simulink model "main_sim_noadapt"  (Simulink 7.2)
settings: Solver=ode2  SolverMode=SingleTasking  StartTime=0.0  StopTime=tsim_max  FixedStep=dtsim  RelTol=1e-3
StopFcn:
  | %mkplt
values from neighbouring files (symbols this model uses):
  vel = 128    [do_command_tracking.m]
undefined symbols (not defined in the file or in its folder): accel_cmd, aero_surf_qbar_off, aero_surf_qbar_on, assertion_time, att_cmd_select, att_trim_IC, att_type, att_type_numbers, bb_ellipsoid, bb_params, chi_trim_IC, command_time, compute_all_rate_cols, compute_all_vel_cols, constants, cosA, da_trim_IC, dc_L2W_IC, de_trim_IC, DiscIntNeverNeededParam, dr_trim_IC, dtsim, E_rwy, E_trim_IC, Ed_cmd, Ed_trim_IC, eow_boundary, flag_exsig, full_surf_llim, full_surf_ulim, gain_set, gain_var_struct, gam_cmd_descent, gam_cmd_preflare, gamdot_cmd_descent, gamdot_cmd_flare, gamdot_cmd_preflare, gamma_trim_IC, h_trim_IC, hd_cmd, hd_trim_IC, ideal_vel_Kb, in_exsig_vecin, in_exsig_vecout, in_t_exsig, MACH, MACH_att_fb, MACH_att_int_IC, MACH_att_Kb, MACH_att_Kc, MACH_att_Ki, MACH_gain_mat, MACH_mass_IC, MACH_pos_IC, MACH_pos_int_IC, MACH_pos_Kb, MACH_pos_Kc, MACH_pos_Ki, MACH_pqr_Bmat_IC, MACH_pqr_IC ... (+62)
libraries: simulink x36, utility_lib x34, mach_lib x24, model_lib x13, simulink_need_slupdate x8, models x8
(part 3 of 7)

== system main_sim_noadapt/claw_main/state est/process inputs ==
  u_old : Inport  OutDataType=sfix(16)  OutScaling=2^0
  sensors : Inport  Port=2  OutDataType=sfix(16)  OutScaling=2^0
  Bus Selector2 : BusSelector  OutputSignals=u_meas
  Constant : Constant  Value=0  OutDataType=sfix(16)  OutScaling=2^0
  Multiport Switch1 : MultiPortSwitch  Inputs=2  zeroidx=on  SaturateOnIntegerOverflow=on
  throt : Selector  InputPortWidth=MACH.num_u  IndexOptions=Index vector (dialog)  Indices=MACH.throttle_idx  OutputSizes=1
  use throt estimate from measurement instead of past throt cmd : Assignment  IndexOptions=Index vector (dialog)  Indices=MACH.throttle_idx  OutputSizes=[1 1]
  use_throt_estimate : Constant  Value=use_throt_estimate  OutDataType=sfix(16)  OutScaling=2^0
  zero RCS inputs : Assignment  IndexOptions=Index vector (dialog)  Indices=MACH.rcs_idx  OutputSizes=[1 1]
  u_est : Outport  OutDataType=sfix(16)  OutScaling=2^0
  wires:
  u_old/1 -> use throt estimate from measurement instead of past throt cmd/1, Multiport Switch1/2
  use_throt_estimate/1 -> Multiport Switch1/1
  use throt estimate from measurement instead of past throt cmd/1 -> Multiport Switch1/3
  sensors/1 -> Bus Selector2/1
  Bus Selector2/1 -> throt/1  "<u_meas>"
  Multiport Switch1/1 -> zero RCS inputs/1
  Constant/1 -> zero RCS inputs/2
  zero RCS inputs/1 -> u_est/1
  throt/1 -> use throt estimate from measurement instead of past throt cmd/2

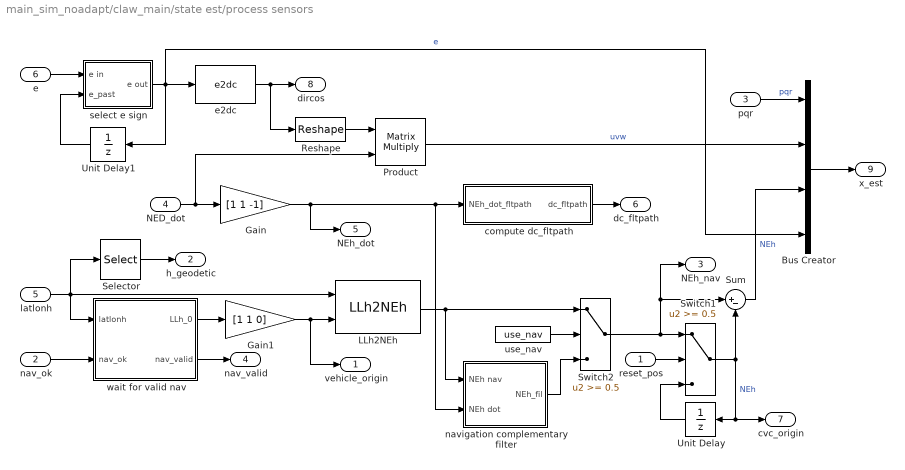
== system main_sim_noadapt/claw_main/state est/process sensors ==
  reset_pos : Inport  OutDataType=sfix(16)  OutScaling=2^0
  nav_ok : Inport  Port=2  OutDataType=sfix(16)  OutScaling=2^0
  pqr : Inport  Port=3  OutDataType=sfix(16)  OutScaling=2^0
  NED_dot : Inport  Port=4  OutDataType=sfix(16)  OutScaling=2^0
  latlonh : Inport  Port=5  OutDataType=sfix(16)  OutScaling=2^0
  e : Inport  Port=6  OutDataType=sfix(16)  OutScaling=2^0
  Bus Creator : BusCreator
  Gain : Gain  Gain=[1 1 -1]  ParameterDataType=sfix(16)  ParameterScaling=2^0  OutDataType=sfix(16)  OutScaling=2^0  SaturateOnIntegerOverflow=on  OutDataTypeStr=Inherit: Same as input  ParamDataTypeStr=Inherit: Same as input
  Gain1 : Gain  Gain=[1 1 0]  ParameterDataType=sfix(16)  ParameterScaling=2^0  OutDataType=sfix(16)  OutScaling=2^0  SaturateOnIntegerOverflow=on  OutDataTypeStr=Inherit: Same as input  ParamDataTypeStr=Inherit: Same as input
  LLh2NEh : utility_lib/LLh2NEh  SystemSampleTime=-1
  Product : Product  Multiplication=Matrix(*)  OutDataType=sfix(16)  OutScaling=2^0  SaturateOnIntegerOverflow=on  OutDataTypeStr=Inherit: Same as first input
  Reshape : Reshape  OutputDimensionality=Customize  OutputDimensions=[3,3]
  Selector : Selector  InputPortWidth=3  IndexOptions=Index vector (dialog)  Indices=[3]  OutputSizes=1
  Sum : Sum  Inputs=|+-  OutDataType=sfix(16)  OutScaling=2^0  SaturateOnIntegerOverflow=on
  Switch1 : Switch  Threshold=0.5  SaturateOnIntegerOverflow=on
  Switch2 : Switch  Threshold=0.5  SaturateOnIntegerOverflow=on
  Unit Delay : UnitDelay  Orientation=left  SampleTime=-1
  Unit Delay1 : UnitDelay  Orientation=left  X0=MACH_quat_IC  SampleTime=-1
  compute dc_fltpath : Subsystem
  e2dc : utility_lib/e2dc  SystemSampleTime=-1
  navigation complementary filter : Subsystem
  select e sign : Subsystem
  use_nav : Constant  Value=use_nav  OutDataType=sfix(16)  OutScaling=2^0
  wait for valid nav : Subsystem
  vehicle_origin : Outport  OutDataType=sfix(16)  OutScaling=2^0
  h_geodetic : Outport  Port=2  OutDataType=sfix(16)  OutScaling=2^0
  NEh_nav : Outport  Port=3  OutDataType=sfix(16)  OutScaling=2^0
  nav_valid : Outport  Port=4  OutDataType=sfix(16)  OutScaling=2^0
  NEh_dot : Outport  Port=5  OutDataType=sfix(16)  OutScaling=2^0
  dc_fltpath : Outport  Port=6  OutDataType=sfix(16)  OutScaling=2^0
  cvc_origin : Outport  Port=7  OutDataType=sfix(16)  OutScaling=2^0
  dircos : Outport  Port=8  OutDataType=sfix(16)  OutScaling=2^0
  x_est : Outport  Port=9  OutDataType=sfix(16)  OutScaling=2^0
  wires:
  e/1 -> select e sign/1(e in)
  Unit Delay1/1 -> select e sign/2(e_past)
  wait for valid nav/1(LLh_0) -> Gain1/1
  Sum/1 -> Bus Creator/3  "NEh"
  navigation complementary filter/1(NEh_fil) -> Switch2/3
  use_nav/1 -> Switch2/2
  Switch2/1 -> Sum/1, NEh_nav/1, Switch1/1
  Unit Delay/1 -> Switch1/3
  Switch1/1 -> Unit Delay/1, cvc_origin/1, Sum/2  "NEh"
  LLh2NEh/1 -> navigation complementary filter/1(NEh nav), Switch2/1
  wait for valid nav/2(nav_valid) -> nav_valid/1
  nav_ok/1 -> wait for valid nav/2(nav_ok)
  reset_pos/1 -> Switch1/2
  latlonh/1 -> wait for valid nav/1(latlonh), LLh2NEh/1, Selector/1
  e2dc/1 -> dircos/1, Reshape/1
  NED_dot/1 -> Product/2, Gain/1
  Gain/1 -> navigation complementary filter/2(NEh dot), compute dc_fltpath/1(NEh_dot_fltpath), NEh_dot/1
  select e sign/1(e out) -> Unit Delay1/1, e2dc/1, Bus Creator/4  "e"
  Reshape/1 -> Product/1
  pqr/1 -> Bus Creator/1  "pqr"
  Product/1 -> Bus Creator/2  "uvw"
  Bus Creator/1 -> x_est/1
  Selector/1 -> h_geodetic/1
  Gain1/1 -> LLh2NEh/2, vehicle_origin/1
  compute dc_fltpath/1(dc_fltpath) -> dc_fltpath/1

== system main_sim_noadapt/claw_main/state est/wind estimator ==
  dircos : Inport  OutDataType=sfix(16)  OutScaling=2^0
  x : Inport  Port=2  OutDataType=sfix(16)  OutScaling=2^0
  sensors : Inport  Port=3  OutDataType=sfix(16)  OutScaling=2^0
  u : Inport  Port=4  OutDataType=sfix(16)  OutScaling=2^0
  wind_est_sw : Inport  Port=5  OutDataType=sfix(16)  OutScaling=2^0
  Bus Selector1 : BusSelector  OutputSignals=NED_wind,accels_cg
  Bus Selector2 : BusSelector  OutputSignals=accels_cg
  Multiport Switch1 : MultiPortSwitch  Inputs=2  zeroidx=on  SaturateOnIntegerOverflow=on
  Unit Delay : UnitDelay  X0=zeros(3,1)  SampleTime=-1
  cl model : models/gtm-obac  SystemSampleTime=-1
  use_wind_est : Constant  Value=use_wind_est  OutDataType=sfix(16)  OutScaling=2^0
  wind estimate : Subsystem
  w_est : Outport  OutDataType=sfix(16)  OutScaling=2^0
  w_est_debug : Outport  Port=2  OutDataType=sfix(16)  OutScaling=2^0
  wires:
  cl model/1 -> wind estimate/3(xdot)
  Unit Delay/1 -> cl model/3
  use_wind_est/1 -> Multiport Switch1/1
  wind estimate/1(w_est) -> Unit Delay/1, Multiport Switch1/3
  x/1 -> wind estimate/2(x), cl model/1
  u/1 -> cl model/2
  dircos/1 -> wind estimate/1(dircos)
  Multiport Switch1/1 -> w_est/1
  wind_est_sw/1 -> wind estimate/6(wind_est_sw)
  sensors/1 -> Bus Selector1/1
  wind estimate/2(w_est_debug) -> w_est_debug/1
  Bus Selector1/1 -> Multiport Switch1/2  "<NED_wind>"
  Bus Selector1/2 -> wind estimate/5(sensed_accels_cg)  "<accels_cg>"
  cl model/2 -> Bus Selector2/1
  Bus Selector2/1 -> wind estimate/4(model_accels_cg)  "<accels_cg>"

== system main_sim_noadapt/claw_main/vel_loops/B matrix comp ==
  note: Note: Ideally,  X_nom and U_nom
      |  would be constructed to be near
      |  moment equalibrium
  X : Inport  OutDataType=sfix(16)  OutScaling=2^0
  U_limited : Inport  Port=2  OutDataType=sfix(16)  OutScaling=2^0
  d_nom : Inport  Port=3  OutDataType=sfix(16)  OutScaling=2^0
  camcmd : Inport  Port=4  OutDataType=sfix(16)  OutScaling=2^0
  params : Inport  Port=5  OutDataType=sfix(16)  OutScaling=2^0
  w_est : Inport  Port=6  OutDataType=sfix(16)  OutScaling=2^0
  NEh_dot : Inport  Port=7  OutDataType=sfix(16)  OutScaling=2^0
  scoped_bus : Inport  Port=8  OutDataType=sfix(16)  OutScaling=2^0
  B matrix comp : Subsystem  TreatAsAtomicUnit=on
  Constant : Constant  Value=0  OutDataType=sfix(16)  OutScaling=2^0
  Constant1 : Constant  Value=0  OutDataType=sfix(16)  OutScaling=2^0
  compute cvd_nom : Subsystem
  compute nominal XU : Subsystem
  zero pqr : Assignment  IndexOptions=Index vector (dialog)  Indices=MACH.pqr_idx  OutputSizes=[1 1]
  zero rate surfs : Assignment  IndexOptions=Index vector (dialog)  Indices=MACH.pqr_u_idx  OutputSizes=[1 1]
  cvd_nom : Outport  OutDataType=sfix(16)  OutScaling=2^0
  Bmat : Outport  Port=2  OutDataType=sfix(16)  OutScaling=2^0
  wires:
  camcmd/1 -> B matrix comp/6(camcmd), compute nominal XU/4(camcmd)
  scoped_bus/1 -> B matrix comp/9(scoped_bus)
  d_nom/1 -> B matrix comp/5(d_nom), compute nominal XU/3(D_in)
  params/1 -> B matrix comp/8(params)
  NEh_dot/1 -> B matrix comp/7(NEh_dot), compute nominal XU/5(NEh_dot)
  compute cvd_nom/1(cvd) -> cvd_nom/1, B matrix comp/1(cvd_nom)
  w_est/1 -> B matrix comp/4(w_est), compute cvd_nom/3(w_est)
  B matrix comp/1(Bmat) -> Bmat/1
  compute nominal XU/1(X_out) -> compute cvd_nom/1(x), B matrix comp/2(X_nom)
  compute nominal XU/2(U_out) -> compute cvd_nom/2(u), B matrix comp/3(U_nom)
  zero rate surfs/1 -> compute nominal XU/2(U_in)
  zero pqr/1 -> compute nominal XU/1(X_in)
  Constant/1 -> zero pqr/2
  Constant1/1 -> zero rate surfs/2
  U_limited/1 -> zero rate surfs/1
  X/1 -> zero pqr/1

== system main_sim_noadapt/claw_main/vel_loops/compute trim ==
  inner cmd : Inport  OutDataType=sfix(16)  OutScaling=2^0
  Bmat : Inport  Port=2  OutDataType=sfix(16)  OutScaling=2^0
  cmd : Inport  Port=3  OutDataType=sfix(16)  OutScaling=2^0
  Product : Product  Multiplication=Matrix(*)  OutDataType=sfix(16)  OutScaling=2^0  SaturateOnIntegerOverflow=on  OutDataTypeStr=Inherit: Same as first input
  Sum1 : Sum  Inputs=|+-  OutDataType=sfix(16)  OutScaling=2^0  SaturateOnIntegerOverflow=on
  trim : Outport  OutDataType=sfix(16)  OutScaling=2^0
  wires:
  Product/1 -> trim/1
  Bmat/1 -> Product/1
  Sum1/1 -> Product/2
  inner cmd/1 -> Sum1/1
  cmd/1 -> Sum1/2

== system main_sim_noadapt/claw_main/vel_loops/config_di ==
  cvd_nom : Inport  OutDataType=sfix(16)  OutScaling=2^0
  Bmat : Inport  Port=2  OutDataType=sfix(16)  OutScaling=2^0
  d_old : Inport  Port=3  OutDataType=sfix(16)  OutScaling=2^0
  d_nom : Inport  Port=4  OutDataType=sfix(16)  OutScaling=2^0
  cvd_des : Inport  Port=5  OutDataType=sfix(16)  OutScaling=2^0
  params : Inport  Port=6  OutDataType=sfix(16)  OutScaling=2^0
  di_smn : mach_lib/di_smn  SystemSampleTime=-1
  d_cmd : Outport  OutDataType=sfix(16)  OutScaling=2^0
  cvd_extra : Outport  Port=2  OutDataType=sfix(16)  OutScaling=2^0
  lambda : Outport  Port=3  OutDataType=sfix(16)  OutScaling=2^0
  solve_dat : Outport  Port=4  OutDataType=sfix(16)  OutScaling=2^0
  wires:
  cvd_nom/1 -> di_smn/1
  Bmat/1 -> di_smn/2
  d_old/1 -> di_smn/3
  d_nom/1 -> di_smn/4
  cvd_des/1 -> di_smn/5
  params/1 -> di_smn/6
  di_smn/1 -> d_cmd/1
  di_smn/2 -> cvd_extra/1
  di_smn/3 -> lambda/1
  di_smn/4 -> solve_dat/1

== system main_sim_noadapt/claw_main/vel_loops/convert accel_cmd to NED_dd_cmd ==
  accel_cmd : Inport  OutDataType=sfix(16)  OutScaling=2^0
  accel_cmd_sw : Inport  Port=2  OutDataType=sfix(16)  OutScaling=2^0
  NEh_d : Inport  Port=3  OutDataType=sfix(16)  OutScaling=2^0
  Merge : Merge  InitialOutput=zeros(3,1)
  MinMax : MinMax  Function=max  OutDataType=sfix(16)  OutScaling=2^0
  NED_dd cmd : Subsystem  TreatAsAtomicUnit=on
  Switch Case : SwitchCase  CaseConditions={1,2}  CaseShowDefault=off
  vchigam_dot cmd : Subsystem  TreatAsAtomicUnit=on
  NEh_dd_cmd : Outport  OutDataType=sfix(16)  OutScaling=2^0
  wires:
  accel_cmd_sw/1 -> MinMax/1
  MinMax/1 -> Switch Case/1
  NEh_d/1 -> vchigam_dot cmd/2(NEh_d)
  vchigam_dot cmd/1(NEh_dd_cmd) -> Merge/2
  Merge/1 -> NEh_dd_cmd/1
  Switch Case/1 -> NED_dd cmd/Action
  Switch Case/2 -> vchigam_dot cmd/Action
  accel_cmd/1 -> vchigam_dot cmd/1(vchigam_dot_cmd), NED_dd cmd/1(NEH_dd_cmd_in)
  NED_dd cmd/1(NEh_dd_cmd) -> Merge/1

== system main_sim_noadapt/claw_main/vel_loops/from inner ==
  att,T : Inport  OutDataType=sfix(16)  OutScaling=2^0
  Demux1 : Demux  Outputs=[ 2 1 MACH.num_u_throt ]
  Mux1 : Mux  Inputs=2
  Terminator : Terminator
  d_cmd : Outport  OutDataType=sfix(16)  OutScaling=2^0
  wires:
  att,T/1 -> Demux1/1
  Demux1/1 -> Mux1/1
  Mux1/1 -> d_cmd/1
  Demux1/3 -> Mux1/2
  Demux1/2 -> Terminator/1

== system main_sim_noadapt/claw_main/vel_loops/from quat ==
  e,T : Inport  OutDataType=sfix(16)  OutScaling=2^0
  Demux1 : Demux  Outputs=[ 4 MACH.num_u_throt ]
  Mux1 : Mux  Inputs=2
  Selector1 : Selector  InputPortWidth=3  IndexOptions=Index vector (dialog)  Indices=1:2  OutputSizes=1
  e2att : utility_lib/e2att  SystemSampleTime=-1
  d_cmd : Outport  OutDataType=sfix(16)  OutScaling=2^0
  wires:
  e2att/1 -> Selector1/1
  Selector1/1 -> Mux1/1
  Demux1/2 -> Mux1/2
  Mux1/1 -> d_cmd/1
  Demux1/1 -> e2att/1
  e,T/1 -> Demux1/1

== system main_sim_noadapt/claw_main/vel_loops/select vel cmd ==
  NEh_dot_current : Inport  OutDataType=sfix(16)  OutScaling=2^0
  cam_current : Inport  Port=2  OutDataType=sfix(16)  OutScaling=2^0
  outer cmd : Inport  Port=3  OutDataType=sfix(16)  OutScaling=2^0
  signal_bus : Inport  Port=4  OutDataType=sfix(16)  OutScaling=2^0
  Bus Selector : BusSelector  OutputSignals=cmd_bus.select_cmd.vel,cmd_bus.autopilot_cmd
  Demux3 : Demux  Outputs=[ MACH.vel_num_cv 1 ]
  Multiport Switch : MultiPortSwitch  zeroidx=on  SaturateOnIntegerOverflow=on
  Mux : Mux  Inputs=2
  Selector1 : Selector  InputPortWidth=4  IndexOptions=Index vector (dialog)  Indices=[1 2 4 3]  OutputSizes=1
  Selector2 : Selector  InputPortWidth=4  IndexOptions=Index vector (dialog)  Indices=[1 2 4 3]  OutputSizes=1
  NEh_dot_cmd : Outport  OutDataType=sfix(16)  OutScaling=2^0
  cam_cmd : Outport  Port=2  OutDataType=sfix(16)  OutScaling=2^0
  cmd : Outport  Port=3  OutDataType=sfix(16)  OutScaling=2^0
  wires:
  Multiport Switch/1 -> cmd/1, Selector2/1
  outer cmd/1 -> Multiport Switch/4
  Bus Selector/1 -> Multiport Switch/1  "<vel>"
  Selector2/1 -> Demux3/1
  Demux3/1 -> NEh_dot_cmd/1
  Demux3/2 -> cam_cmd/1
  Mux/1 -> Selector1/1
  NEh_dot_current/1 -> Mux/1
  Selector1/1 -> Multiport Switch/2
  signal_bus/1 -> Bus Selector/1
  Bus Selector/2 -> Multiport Switch/3  "<autopilot_cmd>"
  cam_current/1 -> Mux/2

== system main_sim_noadapt/claw_main/vel_loops/set di params ==
  note: Note: dc_fltpath is now computed from NEh_dot.
      | Switch to recover old computation base on NEh_dot_cmd
  NEh_dot_cmd : Inport  OutDataType=sfix(16)  OutScaling=2^0
  full_surf : Inport  Port=2  OutDataType=sfix(16)  OutScaling=2^0
  u_old : Inport  Port=3  OutDataType=sfix(16)  OutScaling=2^0
  uvw : Inport  Port=4  OutDataType=sfix(16)  OutScaling=2^0
  dc_fltpath : Inport  Port=5  OutDataType=sfix(16)  OutScaling=2^0
  Bus Creator1 : BusCreator  Inputs=7
  Bus Selector : BusSelector  OutputSignals=u_ulim,u_llim,u_urlim,u_lrlim
  Bus Selector1 : BusSelector  OutputSignals=throt_ulim,throt_llim
  Constant1 : Constant  Value=MACH.vel_wght_cv  OutDataType=sfix(16)  OutScaling=2^0
  Constant3 : Constant  Value=MACH.vel_u_pref  OutDataType=sfix(16)  OutScaling=2^0
  Constant4 : Constant  Value=MACH.vel_wght_u_pref  OutDataType=sfix(16)  OutScaling=2^0
  Demux1 : Demux  Outputs=[ 2 MACH.num_u_throt ]
  Gain2 : Gain  Gain=repmat(MACH.vel_wght_fltpath',1,3)  ParameterDataType=sfix(16)  ParameterScaling=2^0  OutDataType=sfix(16)  OutScaling=2^0
  Logical Operator : Logic  Inputs=1  AllPortsSameDT=off  OutDataTypeMode=boolean  OutDataTypeStr=boolean
  Manual Switch : simulink/Signal Routing/Manual Switch  SystemSampleTime=-1  sw=1  action=0  varsize=off
  Multiport Switch2 : MultiPortSwitch  Inputs=2  zeroidx=on
  Relational Operator : RelationalOperator  Operator===  LogicOutDataTypeMode=boolean  OutDataTypeStr=boolean
  Terminator : Terminator
  att limits : Subsystem
  combine limits : Subsystem
  compute dc_fltpath : Subsystem
  throttle limits : Subsystem
  params : Outport  OutDataType=sfix(16)  OutScaling=2^0
  wires:
  Constant4/1 -> Bus Creator1/6  "wght_u_pref"
  Constant3/1 -> Bus Creator1/5  "u_pref"
  Multiport Switch2/1 -> Bus Creator1/7  "wght_cv"
  Constant1/1 -> Multiport Switch2/2
  full_surf/1 -> throttle limits/1(full_surf)
  Bus Selector/1 -> Bus Creator1/1  "<u_ulim>"
  Bus Selector/2 -> Bus Creator1/2  "<u_llim>"
  Bus Selector/4 -> Bus Creator1/4  "<u_lrlim>"
  Bus Creator1/1 -> params/1
  Relational Operator/1 -> Logical Operator/1
  Logical Operator/1 -> Multiport Switch2/1
  uvw/1 -> att limits/1(uvw)
  att limits/1(att_limits) -> combine limits/1(att_limits)
  throttle limits/1(throt_limits) -> combine limits/2(throt_limits), Bus Selector1/1
  combine limits/1(vel_u_limits) -> Bus Selector/1
  Bus Selector/3 -> Bus Creator1/3  "<u_urlim>"
  Bus Selector1/1 -> Relational Operator/1  "<throt_ulim>"
  Bus Selector1/2 -> Relational Operator/2  "<throt_llim>"
  Demux1/2 -> throttle limits/2(throt_old)
  Demux1/1 -> Terminator/1
  u_old/1 -> Demux1/1
  Gain2/1 -> Multiport Switch2/3
  NEh_dot_cmd/1 -> compute dc_fltpath/1(NEh_dot_fltpath)
  Manual Switch/1 -> Gain2/1
  dc_fltpath/1 -> Manual Switch/1
  compute dc_fltpath/1(dc_fltpath) -> Manual Switch/2

== system main_sim_noadapt/claw_main/vel_loops/to full att/e cmd ==
  d_cmd : Inport  OutDataType=sfix(16)  OutScaling=2^0
  cam : Inport  Port=2  OutDataType=sfix(16)  OutScaling=2^0
  Demux : Demux  Outputs=[ 2 MACH.num_u_throt ]
  Mux : Mux  Inputs=2
  Mux1 : Mux  Inputs=2
  Mux4 : Mux  Inputs=2
  att2e : utility_lib/att2e  SystemSampleTime=-1  quat_IC=MACH_quat_IC
  att,T : Outport  OutDataType=sfix(16)  OutScaling=2^0
  e,T : Outport  Port=2  OutDataType=sfix(16)  OutScaling=2^0
  wires:
  Demux/2 -> Mux/2, Mux1/2  "throt"
  Demux/1 -> Mux4/1
  cam/1 -> Mux4/2
  Mux4/1 -> Mux/1, att2e/1  "att"
  d_cmd/1 -> Demux/1
  Mux/1 -> att,T/1
  att2e/1 -> Mux1/1
  Mux1/1 -> e,T/1

== system main_sim_noadapt/claw_main/vel_loops/xu2d ==
  X : Inport  OutDataType=sfix(16)  OutScaling=2^0
  U : Inport  Port=2  OutDataType=sfix(16)  OutScaling=2^0
  params : Inport  Port=3  OutDataType=sfix(16)  OutScaling=2^0
  Assignment : Assignment  IndexOptions=Index vector (dialog)  Indices=MACH.throttle_idx  OutputSizes=[1 1]
  Bus Selector : BusSelector  OutputSignals=u_llim,u_ulim
  Demux : Demux  Outputs=[ 2 1 ]
  MinMax : MinMax  Inputs=2  OutDataType=sfix(16)  OutScaling=2^0  SaturateOnIntegerOverflow=on  InputSameDT=on
  MinMax1 : MinMax  Function=max  Inputs=2  OutDataType=sfix(16)  OutScaling=2^0  SaturateOnIntegerOverflow=on  InputSameDT=on
  Mux : Mux  Inputs=2
  Reshape : Reshape
  Selector1 : Selector  InputPortWidth=MACH.num_x  IndexOptions=Index vector (dialog)  Indices=MACH.quat_idx  OutputSizes=1
  Selector2 : Selector  InputPortWidth=MACH.num_u  IndexOptions=Index vector (dialog)  Indices=MACH.throttle_idx  OutputSizes=1
  Selector3 : Selector  InputPortWidth=MACH.vel_num_u  IndexOptions=Index vector (dialog)  Indices=3:MACH.vel_num_u  OutputSizes=1
  Selector4 : Selector  InputPortWidth=MACH.vel_num_u  IndexOptions=Index vector (dialog)  Indices=3:MACH.vel_num_u  OutputSizes=1
  e2att : utility_lib/e2att  SystemSampleTime=-1
  U_limited : Outport  OutDataType=sfix(16)  OutScaling=2^0
  d_nom : Outport  Port=2  OutDataType=sfix(16)  OutScaling=2^0
  cam : Outport  Port=3  OutDataType=sfix(16)  OutScaling=2^0
  wires:
  Selector1/1 -> e2att/1
  Selector2/1 -> MinMax1/1  "throttle"
  Mux/1 -> d_nom/1
  X/1 -> Selector1/1
  U/1 -> Selector2/1, Assignment/1
  Demux/1 -> Mux/1
  Demux/2 -> cam/1
  params/1 -> Bus Selector/1
  Bus Selector/1 -> Selector3/1  "<u_llim>"
  MinMax1/1 -> MinMax/1
  Bus Selector/2 -> Selector4/1  "<u_ulim>"
  Selector4/1 -> MinMax/2
  Selector3/1 -> MinMax1/2
  MinMax/1 -> Assignment/2, Reshape/1
  Assignment/1 -> U_limited/1
  e2att/1 -> Demux/1
  Reshape/1 -> Mux/2

== system main_sim_noadapt/control input (modified)/Add Excitation/Excitation  Signal ==
  Enable : EnablePort  StatesWhenEnabling=reset  ShowOutputPort=on
  Gain1 : Gain  Gain=180/pi  ParameterDataType=sfix(16)  ParameterScaling=2^0  OutDataType=sfix(16)  OutScaling=2^0
  Gain3 : Gain  Gain=flag_exsig  ParameterDataType=sfix(16)  ParameterScaling=2^0  OutDataType=sfix(16)  OutScaling=2^0
  Lookup Table1 : Lookup  InputValues=in_exsig_vecin  Table=in_exsig_vecout  LookUpMeth=Use Input Above  OutDataType=sfix(16)  OutScaling=2^0
  excitaiton output sig : Scope
      settings: TimeRange=45  YMin=-0.05  YMax=0.05  SaveName=ScopeData5
  excitation input sig : Scope
      settings: TimeRange=45  YMin=15  YMax=22  SaveName=ScopeData10
  int_Kxhat1 : DiscreteIntegrator  ExternalReset=falling  SampleTime=MACH.dt  OutDataType=sfix(16)  OutScaling=2^0  ICPrevOutput=DiscIntNeverNeededParam  ICPrevScaledInput=DiscIntNeverNeededParam
  exsig : Outport  OutDataType=sfix(16)  OutScaling=2^0  OutputWhenDisabled=reset  InitialOutput=0
  wires:
  int_Kxhat1/1 -> excitation input sig/1, Lookup Table1/1
  Enable/1 -> int_Kxhat1/1, int_Kxhat1/2
  Lookup Table1/1 -> Gain3/1
  Gain1/1 -> excitaiton output sig/1
  Gain3/1 -> exsig/1, Gain1/1

== system main_sim_noadapt/control input (modified)/control input/form control input ==
  cmd_bus : Inport  OutDataType=sfix(16)  OutScaling=2^0
  Bus Creator : BusCreator
  Bus Selector4 : BusSelector  OutputSignals=command,full_surf_cmd
  add effector control params : Subsystem
  engine parameters : Subsystem
  mode switches : Subsystem
  select command : Subsystem
  control_input : Outport  OutDataType=sfix(16)  OutScaling=2^0
  wires:
  Bus Creator/1 -> control_input/1
  cmd_bus/1 -> select command/1(cmd_bus)
  mode switches/1(mode_sw) -> Bus Creator/3  "mode_sw"
  engine parameters/1(engines) -> Bus Creator/4  "engines"
  Bus Selector4/2 -> add effector control params/1(full_surf_cmd)  "<full_surf_cmd>"
  add effector control params/1(full_surf) -> Bus Creator/2  "full_surf"
  Bus Selector4/1 -> Bus Creator/1  "<command>"
  select command/1(control_input) -> mode switches/1(control_input), Bus Selector4/1

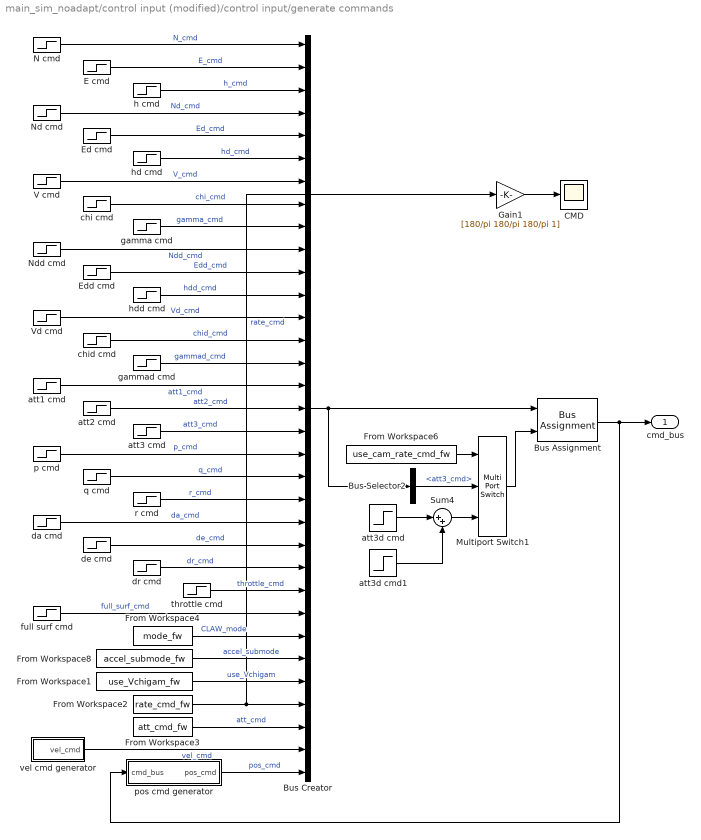
== system main_sim_noadapt/control input (modified)/control input/generate commands ==
  Bus Assignment : BusAssignment  AssignedSignals=att3_cmd
  Bus Creator : BusCreator  Inputs=33
  Bus Selector2 : BusSelector  OutputSignals=att3_cmd
  CMD : Scope
      settings: TimeRange=30  YMax=20  SaveName=ScopeData24
  E cmd : Step  Time=command_time  Before=E_trim_IC  After=E_trim_IC+10*0  SampleTime=MACH.dt
  Ed cmd : Step  Time=command_time  Before=Ed_trim_IC  After=Ed_trim_IC  SampleTime=MACH.dt
  Edd cmd : Step  Time=command_time  After=0  SampleTime=MACH.dt
  From Workspace1 : FromWorkspace  VariableName=use_Vchigam_fw  SampleTime=MACH.dt  Interpolate=off  OutputAfterFinalValue=Holding final value
  From Workspace2 : FromWorkspace  VariableName=rate_cmd_fw  SampleTime=MACH.dt  OutputAfterFinalValue=Holding final value
  From Workspace3 : FromWorkspace  VariableName=att_cmd_fw  SampleTime=MACH.dt  OutputAfterFinalValue=Holding final value
  From Workspace4 : FromWorkspace  VariableName=mode_fw  SampleTime=MACH.dt  Interpolate=off  OutputAfterFinalValue=Holding final value
  From Workspace6 : FromWorkspace  VariableName=use_cam_rate_cmd_fw  SampleTime=MACH.dt  Interpolate=off  OutputAfterFinalValue=Holding final value
  From Workspace8 : FromWorkspace  VariableName=accel_submode_fw  SampleTime=MACH.dt  Interpolate=off  OutputAfterFinalValue=Holding final value
  Gain1 : Gain  Gain=[180/pi 180/pi 180/pi 1]  ParameterDataType=sfix(16)  ParameterScaling=2^0  OutDataType=sfix(16)  OutScaling=2^0
  Multiport Switch1 : MultiPortSwitch  Inputs=2  zeroidx=on
  N cmd : Step  Time=command_time  Before=N_trim_IC  After=N_trim_IC+10*0  SampleTime=MACH.dt
  Nd cmd : Step  Time=command_time  Before=Nd_trim_IC  After=Nd_trim_IC  SampleTime=MACH.dt
  Ndd cmd : Step  Time=command_time  After=0  SampleTime=MACH.dt
  Sum4 : Sum  Inputs=|++  OutDataType=sfix(16)  OutScaling=2^0  SaturateOnIntegerOverflow=on
  V cmd : Step  Time=command_time  Before=V_trim_IC  After=V_trim_IC  SampleTime=MACH.dt
  Vd cmd : Step  Time=command_time  After=0  SampleTime=MACH.dt
  att1 cmd : Step  Tag=mu  Time=command_time  Before=att_trim_IC(1)  After=att_trim_IC(1) + 0.1*0  SampleTime=MACH.dt
      settings: AttributesFormatString=%<Name> (%<Tag>)
  att2 cmd : Step  Tag=alpha  Description=theta  Time=command_time  Before=att_trim_IC(2)  After="att_trim_IC(2)  + 0.1*0"  SampleTime=MACH.dt
      settings: AttributesFormatString=%<Name> (%<Tag>)
  att3 cmd : Step  Tag=beta  Time=command_time  Before=att_trim_IC(3)  After="att_trim_IC(3)  + 0.1*0"  SampleTime=MACH.dt
      settings: AttributesFormatString=%<Name> (%<Tag>)
  att3d cmd : Step  Tag=beta  Time=command_time + (15 - command_time)  After=-0.04*0  SampleTime=MACH.dt
      settings: AttributesFormatString=%<Name> (%<Tag>)
  att3d cmd1 : Step  Time=command_time + (17 - command_time)  After=0.04*0  SampleTime=MACH.dt
  chi cmd : Step  Time=command_time  Before=chi_trim_IC  After=chi_trim_IC  SampleTime=MACH.dt
  chid cmd : Step  Time=command_time  After=0  SampleTime=MACH.dt
  da cmd : Step  Time=command_time  Before=da_trim_IC  After=da_trim_IC  SampleTime=MACH.dt
  de cmd : Step  Time=command_time  Before=de_trim_IC  After=de_trim_IC  SampleTime=MACH.dt
  dr cmd : Step  Time=command_time  Before=dr_trim_IC  After=dr_trim_IC  SampleTime=MACH.dt
  full surf cmd : Step  Time=command_time  Before=MACH_U_nom_IC  After=MACH_U_nom_IC  SampleTime=MACH.dt
  gamma cmd : Step  Time=command_time  Before=gamma_trim_IC  After=gamma_trim_IC  SampleTime=MACH.dt
  gammad cmd : Step  Time=command_time  After=0  SampleTime=MACH.dt
  h cmd : Step  Time=command_time  Before=h_trim_IC  After=h_trim_IC + 10*0  SampleTime=MACH.dt
  hd cmd : Step  Time=command_time  Before=hd_trim_IC  After=hd_trim_IC  SampleTime=MACH.dt
  hdd cmd : Step  Time=command_time  After=0  SampleTime=MACH.dt
  p cmd : Step  Time=command_time  Before=pqr_trim_IC(1)  After=pqr_trim_IC(1) + 0.2*0  SampleTime=MACH.dt
  pos cmd generator : Subsystem
  q cmd : Step  Time=command_time  Before=pqr_trim_IC(2)  After=pqr_trim_IC(2) + 0.2*0  SampleTime=MACH.dt
  r cmd : Step  Time=command_time  Before=pqr_trim_IC(3)  After=pqr_trim_IC(3) + 0.2*0  SampleTime=MACH.dt
  throttle cmd : Step  Time=command_time  Before=throttle_trim_IC(1)  After=throttle_trim_IC(1)  SampleTime=MACH.dt
  vel cmd generator : Subsystem
  cmd_bus : Outport  OutDataType=sfix(16)  OutScaling=2^0
  wires:
  Bus Creator/1 -> Bus Assignment/1, Bus Selector2/1
  throttle cmd/1 -> Bus Creator/25  "throttle_cmd"
  dr cmd/1 -> Bus Creator/24  "dr_cmd"
  de cmd/1 -> Bus Creator/23  "de_cmd"
  da cmd/1 -> Bus Creator/22  "da_cmd"
  r cmd/1 -> Bus Creator/21  "r_cmd"
  q cmd/1 -> Bus Creator/20  "q_cmd"
  p cmd/1 -> Bus Creator/19  "p_cmd"
  att3 cmd/1 -> Bus Creator/18  "att3_cmd"
  att2 cmd/1 -> Bus Creator/17  "att2_cmd"
  att1 cmd/1 -> Bus Creator/16  "att1_cmd"
  hd cmd/1 -> Bus Creator/6  "hd_cmd"
  Ed cmd/1 -> Bus Creator/5  "Ed_cmd"
  Nd cmd/1 -> Bus Creator/4  "Nd_cmd"
  h cmd/1 -> Bus Creator/3  "h_cmd"
  E cmd/1 -> Bus Creator/2  "E_cmd"
  N cmd/1 -> Bus Creator/1  "N_cmd"
  From Workspace6/1 -> Multiport Switch1/1
  Sum4/1 -> Multiport Switch1/3
  att3d cmd/1 -> Sum4/1
  att3d cmd1/1 -> Sum4/2
  Bus Selector2/1 -> Multiport Switch1/2  "<att3_cmd>"
  Multiport Switch1/1 -> Bus Assignment/2
  Bus Assignment/1 -> pos cmd generator/1(cmd_bus), cmd_bus/1
  From Workspace3/1 -> Bus Creator/31  "att_cmd"
  vel cmd generator/1(vel_cmd) -> Bus Creator/32  "vel_cmd"
  pos cmd generator/1(pos_cmd) -> Bus Creator/33  "pos_cmd"
  From Workspace4/1 -> Bus Creator/27  "CLAW_mode"
  From Workspace8/1 -> Bus Creator/28  "accel_submode"
  full surf cmd/1 -> Bus Creator/26  "full_surf_cmd"
  Ndd cmd/1 -> Bus Creator/10  "Ndd_cmd"
  Edd cmd/1 -> Bus Creator/11  "Edd_cmd"
  hdd cmd/1 -> Bus Creator/12  "hdd_cmd"
  Vd cmd/1 -> Bus Creator/13  "Vd_cmd"
  chid cmd/1 -> Bus Creator/14  "chid_cmd"
  gammad cmd/1 -> Bus Creator/15  "gammad_cmd"
  V cmd/1 -> Bus Creator/7  "V_cmd"
  chi cmd/1 -> Bus Creator/8  "chi_cmd"
  gamma cmd/1 -> Bus Creator/9  "gamma_cmd"
  From Workspace1/1 -> Bus Creator/29  "use_Vchigam"
  From Workspace2/1 -> Bus Creator/30, Gain1/1  "rate_cmd"
  Gain1/1 -> CMD/1

== system main_sim_noadapt/control input (modified)/ideal responses/ideal att rate response ==
  control_input : Inport  OutDataType=sfix(16)  OutScaling=2^0
  Bus Selector1 : BusSelector  OutputSignals=mode_sw.att_type
  Discrete-Time Integrator1 : DiscreteIntegrator  InitialCondition=MACH_pqr_IC  SampleTime=-1  OutDataType=sfix(16)  OutScaling=2^0  ICPrevOutput=DiscIntNeverNeededParam  ICPrevScaledInput=DiscIntNeverNeededParam
  Discrete-Time Integrator3 : DiscreteIntegrator  InitialCondition=MACH_quat_IC  SampleTime=-1  OutDataType=sfix(16)  OutScaling=2^0  ICPrevOutput=DiscIntNeverNeededParam  ICPrevScaledInput=DiscIntNeverNeededParam
  Goto Tag Visibility1 : GotoTagVisibility  GotoTag=dc_L2W
  Goto Tag Visibility8 : GotoTagVisibility  GotoTag=att_type
  Mux : Mux  Inputs=2
  Mux1 : Mux  Inputs=2
  Reshape3 : Reshape  OutputDimensions=[3 3]
  Selector : Selector  InputPortWidth=4  IndexOptions=Index vector (dialog)  Indices=[1 2 3]  OutputSizes=1
  Selector2 : Selector  InputPortWidth=8  IndexOptions=Index vector (port)  Indices=[4 5 3]  OutputSizes=1
  Selector3 : Selector  InputPortWidth=6  IndexOptions=Index vector (port)  Indices=[1 2 6]  OutputSizes=1
  Terminator : Terminator
  To Workspace : ToWorkspace  VariableName=ideal_quat  SampleTime=MACH.dt  SaveFormat=Array
  To Workspace1 : ToWorkspace  VariableName=ideal_rpy  SampleTime=MACH.dt  SaveFormat=Array
  To Workspace2 : ToWorkspace  VariableName=ideal_tiltcam  SampleTime=MACH.dt  SaveFormat=Array
  To Workspace3 : ToWorkspace  VariableName=ideal_mab  SampleTime=MACH.dt  SaveFormat=Array
  To Workspace4 : ToWorkspace  VariableName=ideal_pqr  SampleTime=MACH.dt  SaveFormat=Array
  att loop : Subsystem
  dc2mba : utility_lib/dc2mba  SystemSampleTime=-1
  dc2tiltcam : utility_lib/dc2tiltcam  SystemSampleTime=-1
  dc2ypr : utility_lib/dc2ypr  SystemSampleTime=-1
  dc_L2W : Constant  Value=dc_L2W_IC  OutDataType=sfix(16)  OutScaling=2^0
  e2dc : utility_lib/e2dc  SystemSampleTime=-1
  get att cmd : Subsystem
  geted : utility_lib/geted  SystemSampleTime=-1
  rate loop : Subsystem
  tag scope: att_type=scoped, dc_L2W=scoped
  wires:
  Discrete-Time Integrator3/1 -> To Workspace/1, geted/2, e2dc/1, att loop/2(e), Mux/2, get att cmd/2(e)
  geted/1 -> Discrete-Time Integrator3/1
  get att cmd/1(quatpqr_cmd) -> Selector/1, Mux/1
  rate loop/1(pqrdot) -> Discrete-Time Integrator1/1
  dc_L2W/1 -> Reshape3/1
  Reshape3/1 -> [dc_L2W]
  [dc_L2W] -> Terminator/1
  e2dc/1 -> dc2ypr/1, dc2mba/1, dc2tiltcam/1
  dc2tiltcam/1 -> To Workspace2/1
  dc2ypr/1 -> To Workspace1/1
  dc2mba/1 -> To Workspace3/1
  control_input/1 -> get att cmd/1(control_input), Bus Selector1/1
  Discrete-Time Integrator1/1 -> geted/1, rate loop/2(pqr), To Workspace4/1
  Selector3/1 -> rate loop/1(pqr_cmd)
  Mux1/1 -> Selector3/1
  att loop/1(pqr_cmd) -> Mux1/2
  Selector/1 -> Mux1/1
  get att cmd/3(pqr_select) -> Selector3/2
  Selector2/1 -> att loop/1(e_cmd)
  Mux/1 -> Selector2/1
  get att cmd/2(quat_select) -> Selector2/2
  Bus Selector1/1 -> [att_type]  "<att_type>"

== system main_sim_noadapt/control input (modified)/ideal responses/ideal pos vel response ==
  note: Note: If pos cv is is shifted to zero, add pos_IC after feedback pickoff.
      | If pos cv is real position values, set integrator IC to pos_IC
  control_input : Inport  OutDataType=sfix(16)  OutScaling=2^0
  Constant4 : Constant  Value=MACH_pos_IC*0  OutDataType=sfix(16)  OutScaling=2^0
  Discrete-Time Integrator1 : DiscreteIntegrator  InitialCondition=MACH_vel_IC  SampleTime=-1  OutDataType=sfix(16)  OutScaling=2^0  ICPrevOutput=DiscIntNeverNeededParam  ICPrevScaledInput=DiscIntNeverNeededParam
  Discrete-Time Integrator3 : DiscreteIntegrator  InitialCondition=MACH_pos_IC  SampleTime=-1  OutDataType=sfix(16)  OutScaling=2^0  ICPrevOutput=DiscIntNeverNeededParam  ICPrevScaledInput=DiscIntNeverNeededParam
  Mux : Mux  Inputs=2
  Mux1 : Mux  Inputs=2
  Selector2 : Selector  InputPortWidth=6  IndexOptions=Index vector (port)  Indices=[4 5 3]  OutputSizes=1
  Selector3 : Selector  InputPortWidth=6  IndexOptions=Index vector (port)  Indices=[1 2 6]  OutputSizes=1
  Sum1 : Sum  Inputs=++|  OutDataType=sfix(16)  OutScaling=2^0  SaturateOnIntegerOverflow=on  InputSameDT=on  OutDataTypeStr=Inherit: Same as first input
  To Workspace : ToWorkspace  VariableName=ideal_pos  SampleTime=MACH.dt  SaveFormat=Array
  To Workspace1 : ToWorkspace  VariableName=ideal_vel  SampleTime=MACH.dt  SaveFormat=Array
  get posvel cmd : Subsystem
  pos loop : Subsystem
  vel loop : Subsystem
  wires:
  Discrete-Time Integrator3/1 -> Sum1/2, pos loop/2(NEh), Mux/2
  Mux/1 -> Selector2/1
  vel loop/1(NEhdotdot) -> Discrete-Time Integrator1/1
  Sum1/1 -> To Workspace/1
  Constant4/1 -> Sum1/1
  Selector3/1 -> vel loop/1(NEhdot_cmd)
  pos loop/1(NEhdot_cmd) -> Mux1/2
  get posvel cmd/1(posvel_cmd) -> Mux/1, Mux1/1  "NEh"
  Mux1/1 -> Selector3/1
  control_input/1 -> get posvel cmd/1(control_input)
  get posvel cmd/3(vel_select) -> Selector3/2
  get posvel cmd/2(pos_select) -> Selector2/2
  Selector2/1 -> pos loop/1(NEh_cmd)
  Discrete-Time Integrator1/1 -> Discrete-Time Integrator3/1, To Workspace1/1, vel loop/2(NEhdot)

== system main_sim_noadapt/vehicle_model/target/seeker model/seeker model ==
  NEh_target : Inport  OutDataType=sfix(16)  OutScaling=2^0
  NEh_d_target : Inport  Port=2  OutDataType=sfix(16)  OutScaling=2^0
  NEh : Inport  Port=3  OutDataType=sfix(16)  OutScaling=2^0
  NEh_d : Inport  Port=4  OutDataType=sfix(16)  OutScaling=2^0
  Bus Creator : BusCreator  Inputs=2
  Product1 : Product  Multiplication=Matrix(*)  OutDataType=sfix(16)  OutScaling=2^0  RndMeth=Zero
  Reshape : Reshape  OutputDimensionality=Customize  OutputDimensions=[3 3]
  Selector : Selector  NumberOfDimensions=2  InputPortWidth=3  IndexOptions=Index vector (dialog),Select all  Indices=2:3,-1  OutputSizes=1
  Sum : Sum  Inputs=|+-  OutDataType=sfix(16)  OutScaling=2^0
  Sum1 : Sum  Inputs=|+-  OutDataType=sfix(16)  OutScaling=2^0
  cart to polar : Subsystem
  convert to NED : Gain  Gain=[1 1 -1]  ParameterDataType=sfix(16)  ParameterScaling=2^0  OutDataType=sfix(16)  OutScaling=2^0
  convert to NED_d : Gain  Gain=[1 1 -1]  ParameterDataType=sfix(16)  ParameterScaling=2^0  OutDataType=sfix(16)  OutScaling=2^0
  vec2dc : utility_lib/vec2dc  SystemSampleTime=-1
  seeker : Outport  OutDataType=sfix(16)  OutScaling=2^0
  wires:
  cart to polar/1(LOS_rate) -> Bus Creator/1  "LOS_rate"
  NEh_d_target/1 -> Sum1/1
  NEh_target/1 -> Sum/1
  NEh_d/1 -> Sum1/2
  NEh/1 -> Sum/2
  convert to NED_d/1 -> Product1/2
  Product1/1 -> cart to polar/2(cross_d;vert_d)
  Sum1/1 -> convert to NED_d/1
  Selector/1 -> Product1/1
  convert to NED/1 -> vec2dc/1
  Sum/1 -> convert to NED/1
  Reshape/1 -> Selector/1
  vec2dc/1 -> Reshape/1
  vec2dc/2 -> cart to polar/1(scaling info), Bus Creator/2  "aux_info"
  Bus Creator/1 -> seeker/1

== system main_sim_noadapt/claw_main/att_loops/dyn inv/Limit rate cmd ==
  limit_pqr_cmd : Inport  OutDataType=sfix(16)  OutScaling=2^0
  uvw : Inport  Port=2  OutDataType=sfix(16)  OutScaling=2^0
  pqr : Inport  Port=3  OutDataType=sfix(16)  OutScaling=2^0
  Constant1 : Constant  Value=MACH.az_llim  OutDataType=sfix(16)  OutScaling=2^0
  Constant2 : Constant  Value=MACH.att_u_llim  OutDataType=sfix(16)  OutScaling=2^0
  Constant3 : Constant  Value=MACH.att_u_ulim  OutDataType=sfix(16)  OutScaling=2^0
  Constant4 : Constant  Value=MACH.az_ulim  OutDataType=sfix(16)  OutScaling=2^0
  Enforce lower limit : MinMax  Function=max  Inputs=2  OutDataType=sfix(16)  OutScaling=2^-10  OutDataTypeStr=Inherit: Inherit via back propagation  ZeroCross=off
  Enforce upper limit : MinMax  Inputs=2  OutDataType=sfix(16)  OutScaling=2^-10  OutDataTypeStr=Inherit: Inherit via back propagation  ZeroCross=off
  Multiport Switch : MultiPortSwitch  Inputs=2  zeroidx=on
  velocity based angular rate llim : mach_lib/velocity based angular rate limit  SystemSampleTime=-1  q_idx=2
  velocity based angular rate ulim : mach_lib/velocity based angular rate limit  SystemSampleTime=-1  q_idx=2
  pqr_limited : Outport  OutDataType=sfix(16)  OutScaling=2^0
  wires:
  Enforce lower limit/1 -> Enforce upper limit/1
  pqr/1 -> Enforce lower limit/1, Multiport Switch/2
  velocity based angular rate ulim/1 -> Enforce upper limit/2
  uvw/1 -> velocity based angular rate ulim/3, velocity based angular rate llim/3
  Constant2/1 -> velocity based angular rate llim/1
  Constant4/1 -> velocity based angular rate llim/2
  Constant1/1 -> velocity based angular rate ulim/2
  Constant3/1 -> velocity based angular rate ulim/1  "upper_limit"
  velocity based angular rate llim/1 -> Enforce lower limit/2
  Enforce upper limit/1 -> Multiport Switch/3
  Multiport Switch/1 -> pqr_limited/1
  limit_pqr_cmd/1 -> Multiport Switch/1

== system main_sim_noadapt/claw_main/att_loops/select att cmd/get direct cmd ==
  signal_bus : Inport  OutDataType=sfix(16)  OutScaling=2^0
  Bus Selector : BusSelector  OutputSignals=cmd_bus.autopilot_cmd,mode_sw.full_surf_cmd_sw,full_surf.full_surf_cmd
  Demux1 : Demux  Outputs=[ 3 1 ]
  Gain : Gain  Gain=MACH.throt_mixer  ParameterDataType=sfix(16)  ParameterScaling=2^0  OutDataType=sfix(16)  OutScaling=2^0
  Multiport Switch2 : MultiPortSwitch  Inputs=2  zeroidx=on
  throttle : Selector  InputPortWidth=MACH.num_u  IndexOptions=Index vector (dialog)  Indices=MACH.throttle_idx  OutputSizes=1
  att : Outport  OutDataType=sfix(16)  OutScaling=2^0
  throt : Outport  Port=2  OutDataType=sfix(16)  OutScaling=2^0
  wires:
  Demux1/1 -> att/1
  Demux1/2 -> Gain/1
  signal_bus/1 -> Bus Selector/1
  Bus Selector/1 -> Demux1/1  "<autopilot_cmd>"
  Bus Selector/2 -> Multiport Switch2/1  "<full_surf_cmd_sw>"
  Gain/1 -> Multiport Switch2/2
  Bus Selector/3 -> throttle/1  "<full_surf_cmd>"
  throttle/1 -> Multiport Switch2/3
  Multiport Switch2/1 -> throt/1

== system main_sim_noadapt/claw_main/grab ExportedGlobal/grab cv variables/Subsystem ==
  In1 : Inport  OutDataType=sfix(16)  OutScaling=2^0
  In2 : Inport  Port=2  OutDataType=sfix(16)  OutScaling=2^0
  In3 : Inport  Port=3  OutDataType=sfix(16)  OutScaling=2^0
  In4 : Inport  Port=4  OutDataType=sfix(16)  OutScaling=2^0
  In5 : Inport  Port=5  OutDataType=sfix(16)  OutScaling=2^0
  In6 : Inport  Port=6  OutDataType=sfix(16)  OutScaling=2^0
  In7 : Inport  Port=7  OutDataType=sfix(16)  OutScaling=2^0
  In8 : Inport  Port=8  OutDataType=sfix(16)  OutScaling=2^0
  In9 : Inport  Port=9  OutDataType=sfix(16)  OutScaling=2^0
  In10 : Inport  Port=10  OutDataType=sfix(16)  OutScaling=2^0
  In11 : Inport  Port=11  OutDataType=sfix(16)  OutScaling=2^0
  In12 : Inport  Port=12  OutDataType=sfix(16)  OutScaling=2^0
  In13 : Inport  Port=13  OutDataType=sfix(16)  OutScaling=2^0
  Out1 : Outport  OutDataType=sfix(16)  OutScaling=2^0
  Out2 : Outport  Port=2  OutDataType=sfix(16)  OutScaling=2^0
  Out3 : Outport  Port=3  OutDataType=sfix(16)  OutScaling=2^0
  Out4 : Outport  Port=4  OutDataType=sfix(16)  OutScaling=2^0
  Out5 : Outport  Port=5  OutDataType=sfix(16)  OutScaling=2^0
  Out6 : Outport  Port=6  OutDataType=sfix(16)  OutScaling=2^0
  Out7 : Outport  Port=7  OutDataType=sfix(16)  OutScaling=2^0
  Out8 : Outport  Port=8  OutDataType=sfix(16)  OutScaling=2^0
  Out9 : Outport  Port=9  OutDataType=sfix(16)  OutScaling=2^0
  Out10 : Outport  Port=10  OutDataType=sfix(16)  OutScaling=2^0
  Out11 : Outport  Port=11  OutDataType=sfix(16)  OutScaling=2^0
  Out12 : Outport  Port=12  OutDataType=sfix(16)  OutScaling=2^0
  Out13 : Outport  Port=13  OutDataType=sfix(16)  OutScaling=2^0
  wires:
  In1/1 -> Out1/1
  In2/1 -> Out2/1
  In3/1 -> Out3/1
  In4/1 -> Out4/1
  In5/1 -> Out5/1
  In6/1 -> Out6/1
  In7/1 -> Out7/1
  In8/1 -> Out8/1
  In9/1 -> Out9/1
  In10/1 -> Out10/1
  In11/1 -> Out11/1
  In12/1 -> Out12/1
  In13/1 -> Out13/1

== system main_sim_noadapt/claw_main/grab ExportedGlobal/grab cvcmd variables/Subsystem ==
  In1 : Inport  OutDataType=sfix(16)  OutScaling=2^0
  In2 : Inport  Port=2  OutDataType=sfix(16)  OutScaling=2^0
  In3 : Inport  Port=3  OutDataType=sfix(16)  OutScaling=2^0
  In4 : Inport  Port=4  OutDataType=sfix(16)  OutScaling=2^0
  In5 : Inport  Port=5  OutDataType=sfix(16)  OutScaling=2^0
  In6 : Inport  Port=6  OutDataType=sfix(16)  OutScaling=2^0
  In7 : Inport  Port=7  OutDataType=sfix(16)  OutScaling=2^0
  In8 : Inport  Port=8  OutDataType=sfix(16)  OutScaling=2^0
  In9 : Inport  Port=9  OutDataType=sfix(16)  OutScaling=2^0
  In10 : Inport  Port=10  OutDataType=sfix(16)  OutScaling=2^0
  In11 : Inport  Port=11  OutDataType=sfix(16)  OutScaling=2^0
  In12 : Inport  Port=12  OutDataType=sfix(16)  OutScaling=2^0
  In13 : Inport  Port=13  OutDataType=sfix(16)  OutScaling=2^0
  Out1 : Outport  OutDataType=sfix(16)  OutScaling=2^0
  Out2 : Outport  Port=2  OutDataType=sfix(16)  OutScaling=2^0
  Out3 : Outport  Port=3  OutDataType=sfix(16)  OutScaling=2^0
  Out4 : Outport  Port=4  OutDataType=sfix(16)  OutScaling=2^0
  Out5 : Outport  Port=5  OutDataType=sfix(16)  OutScaling=2^0
  Out6 : Outport  Port=6  OutDataType=sfix(16)  OutScaling=2^0
  Out7 : Outport  Port=7  OutDataType=sfix(16)  OutScaling=2^0
  Out8 : Outport  Port=8  OutDataType=sfix(16)  OutScaling=2^0
  Out9 : Outport  Port=9  OutDataType=sfix(16)  OutScaling=2^0
  Out10 : Outport  Port=10  OutDataType=sfix(16)  OutScaling=2^0
  Out11 : Outport  Port=11  OutDataType=sfix(16)  OutScaling=2^0
  Out12 : Outport  Port=12  OutDataType=sfix(16)  OutScaling=2^0
  Out13 : Outport  Port=13  OutDataType=sfix(16)  OutScaling=2^0
  wires:
  In1/1 -> Out1/1
  In2/1 -> Out2/1
  In3/1 -> Out3/1
  In4/1 -> Out4/1
  In5/1 -> Out5/1
  In6/1 -> Out6/1
  In7/1 -> Out7/1
  In8/1 -> Out8/1
  In9/1 -> Out9/1
  In10/1 -> Out10/1
  In11/1 -> Out11/1
  In12/1 -> Out12/1
  In13/1 -> Out13/1

== system main_sim_noadapt/claw_main/grab ExportedGlobal/grab cvdex variables/Subsystem ==
  In1 : Inport  OutDataType=sfix(16)  OutScaling=2^0
  In2 : Inport  Port=2  OutDataType=sfix(16)  OutScaling=2^0
  In3 : Inport  Port=3  OutDataType=sfix(16)  OutScaling=2^0
  In4 : Inport  Port=4  OutDataType=sfix(16)  OutScaling=2^0
  In5 : Inport  Port=5  OutDataType=sfix(16)  OutScaling=2^0
  In6 : Inport  Port=6  OutDataType=sfix(16)  OutScaling=2^0
  In7 : Inport  Port=7  OutDataType=sfix(16)  OutScaling=2^0
  In8 : Inport  Port=8  OutDataType=sfix(16)  OutScaling=2^0
  In9 : Inport  Port=9  OutDataType=sfix(16)  OutScaling=2^0
  In10 : Inport  Port=10  OutDataType=sfix(16)  OutScaling=2^0
  In11 : Inport  Port=11  OutDataType=sfix(16)  OutScaling=2^0
  In12 : Inport  Port=12  OutDataType=sfix(16)  OutScaling=2^0
  In13 : Inport  Port=13  OutDataType=sfix(16)  OutScaling=2^0
  Out1 : Outport  OutDataType=sfix(16)  OutScaling=2^0
  Out2 : Outport  Port=2  OutDataType=sfix(16)  OutScaling=2^0
  Out3 : Outport  Port=3  OutDataType=sfix(16)  OutScaling=2^0
  Out4 : Outport  Port=4  OutDataType=sfix(16)  OutScaling=2^0
  Out5 : Outport  Port=5  OutDataType=sfix(16)  OutScaling=2^0
  Out6 : Outport  Port=6  OutDataType=sfix(16)  OutScaling=2^0
  Out7 : Outport  Port=7  OutDataType=sfix(16)  OutScaling=2^0
  Out8 : Outport  Port=8  OutDataType=sfix(16)  OutScaling=2^0
  Out9 : Outport  Port=9  OutDataType=sfix(16)  OutScaling=2^0
  Out10 : Outport  Port=10  OutDataType=sfix(16)  OutScaling=2^0
  Out11 : Outport  Port=11  OutDataType=sfix(16)  OutScaling=2^0
  Out12 : Outport  Port=12  OutDataType=sfix(16)  OutScaling=2^0
  Out13 : Outport  Port=13  OutDataType=sfix(16)  OutScaling=2^0
  wires:
  In1/1 -> Out1/1
  In2/1 -> Out2/1
  In3/1 -> Out3/1
  In4/1 -> Out4/1
  In5/1 -> Out5/1
  In6/1 -> Out6/1
  In7/1 -> Out7/1
  In8/1 -> Out8/1
  In9/1 -> Out9/1
  In10/1 -> Out10/1
  In11/1 -> Out11/1
  In12/1 -> Out12/1
  In13/1 -> Out13/1

== system main_sim_noadapt/claw_main/grab ExportedGlobal/grab integrator variables/Subsystem ==
  In1 : Inport  OutDataType=sfix(16)  OutScaling=2^0
  In2 : Inport  Port=2  OutDataType=sfix(16)  OutScaling=2^0
  In3 : Inport  Port=3  OutDataType=sfix(16)  OutScaling=2^0
  In4 : Inport  Port=4  OutDataType=sfix(16)  OutScaling=2^0
  In5 : Inport  Port=5  OutDataType=sfix(16)  OutScaling=2^0
  In6 : Inport  Port=6  OutDataType=sfix(16)  OutScaling=2^0
  In7 : Inport  Port=7  OutDataType=sfix(16)  OutScaling=2^0
  In8 : Inport  Port=8  OutDataType=sfix(16)  OutScaling=2^0
  In9 : Inport  Port=9  OutDataType=sfix(16)  OutScaling=2^0
  In10 : Inport  Port=10  OutDataType=sfix(16)  OutScaling=2^0
  In11 : Inport  Port=11  OutDataType=sfix(16)  OutScaling=2^0
  In12 : Inport  Port=12  OutDataType=sfix(16)  OutScaling=2^0
  In13 : Inport  Port=13  OutDataType=sfix(16)  OutScaling=2^0
  Out1 : Outport  OutDataType=sfix(16)  OutScaling=2^0
  Out2 : Outport  Port=2  OutDataType=sfix(16)  OutScaling=2^0
  Out3 : Outport  Port=3  OutDataType=sfix(16)  OutScaling=2^0
  Out4 : Outport  Port=4  OutDataType=sfix(16)  OutScaling=2^0
  Out5 : Outport  Port=5  OutDataType=sfix(16)  OutScaling=2^0
  Out6 : Outport  Port=6  OutDataType=sfix(16)  OutScaling=2^0
  Out7 : Outport  Port=7  OutDataType=sfix(16)  OutScaling=2^0
  Out8 : Outport  Port=8  OutDataType=sfix(16)  OutScaling=2^0
  Out9 : Outport  Port=9  OutDataType=sfix(16)  OutScaling=2^0
  Out10 : Outport  Port=10  OutDataType=sfix(16)  OutScaling=2^0
  Out11 : Outport  Port=11  OutDataType=sfix(16)  OutScaling=2^0
  Out12 : Outport  Port=12  OutDataType=sfix(16)  OutScaling=2^0
  Out13 : Outport  Port=13  OutDataType=sfix(16)  OutScaling=2^0
  wires:
  In1/1 -> Out1/1
  In2/1 -> Out2/1
  In3/1 -> Out3/1
  In4/1 -> Out4/1
  In5/1 -> Out5/1
  In6/1 -> Out6/1
  In7/1 -> Out7/1
  In8/1 -> Out8/1
  In9/1 -> Out9/1
  In10/1 -> Out10/1
  In11/1 -> Out11/1
  In12/1 -> Out12/1
  In13/1 -> Out13/1

== system main_sim_noadapt/claw_main/grab ExportedGlobal/grab w_est variables/Subsystem ==
  In1 : Inport  OutDataType=sfix(16)  OutScaling=2^0
  In2 : Inport  Port=2  OutDataType=sfix(16)  OutScaling=2^0
  In3 : Inport  Port=3  OutDataType=sfix(16)  OutScaling=2^0
  Out1 : Outport  OutDataType=sfix(16)  OutScaling=2^0
  Out2 : Outport  Port=2  OutDataType=sfix(16)  OutScaling=2^0
  Out3 : Outport  Port=3  OutDataType=sfix(16)  OutScaling=2^0
  wires:
  In1/1 -> Out1/1
  In2/1 -> Out2/1
  In3/1 -> Out3/1
